simulink model "RS_O_yalmip"  (R2016b)
settings: Solver=ode1  StartTime=0.0  StopTime=T  FixedStep=1e-4  MaxStep=1e-3  RelTol=1e-6  EnableMultiTasking=on
InitFcn:
  | RS_O_script;
values from neighbouring files (symbols this model uses):
  C1 = 1e-9    (= 1e-09)    [Dati_MPC.m]
  C2 = 1e-9    (= 1e-09)    [Dati_MPC.m]
  Cext_Bp1 = Ce_Bp1*np_Bp1/ns_Bp1    (= 35750)    [Dati_MPC.m]
  Cext_Bp2 = Ce_Bp2*np_Bp2/ns_Bp2    (= 35750)    [Dati_MPC.m]
  Cext_BpM = Ce_BpM*np_BpM/ns_BpM    (= 68250)    [Dati_MPC.m]
  Cin_Bp1 = Ci_Bp1*np_Bp1/ns_Bp1    (= 16500)    [Dati_MPC.m]
  Cin_Bp2 = Ci_Bp2*np_Bp2/ns_Bp2    (= 16500)    [Dati_MPC.m]
  Cin_BpM = Ci_BpM*np_BpM/ns_BpM    (= 31500)    [Dati_MPC.m]
  Cint = 18e-3    (= 0.018)    [Dati_MPC.m]
  f = 50    [Dati_rete.m]
  ft_F = 10    [Dati_MPC.m]
  I_u = 0.1    [Dati_MPC.m]
  ki_PLL = w_t/Vd*(-w_t+sqrt(2*w_t^2-Vd^2*kp_PLL^2))    [Dati_MPC.m]
  kp_PLL = 0.9*kp_PLL_max    [Dati_MPC.m]
  MPCpar = struct    [Dati_MPC.m]    (also in Initialization.m)
  netdata = struct    [Dati_rete.m]
  P1 = 750e3    (= 750000)    [RS_O_script.m]
  P1v = 500e3    (= 500000)    [RS_O_script.m]
  P2 = 750e3    (= 750000)    [RS_O_script.m]
  P2v = 250e3    (= 250000)    [RS_O_script.m]
  P_u = 0.005    [Dati_MPC.m]
  Ppv1 = 500e3    (= 500000)    [Dati_MPC.m]
  Ppv2 = 850e3    (= 850000)    [Dati_MPC.m]
  Q1 = 350e3    (= 350000)    [RS_O_script.m]
  Q1v = 250e3    (= 250000)    [RS_O_script.m]
  Q2 = 300e3    (= 300000)    [RS_O_script.m]
  Q2v = 250e3    (= 250000)    [RS_O_script.m]
  Qbat1 = 50e3    (= 50000)    [Dati_MPC.m]
  Qbat2 = 50e3    (= 50000)    [Dati_MPC.m]
  Rext_Bp1 = Re_Bp1*ns_Bp1/np_Bp1    (= 0.0154545454545)    [Dati_MPC.m]
  Rext_Bp2 = Re_Bp2*ns_Bp2/np_Bp2    (= 0.0154545454545)    [Dati_MPC.m]
  Rext_BpM = Re_BpM*ns_BpM/np_BpM    (= 0.00809523809524)    [Dati_MPC.m]
  Rin_Bp1 = Ri_Bp1*ns_Bp1/np_Bp1    (= 0.363636363636)    [Dati_MPC.m]
  Rin_Bp2 = Ri_Bp2*ns_Bp2/np_Bp2    (= 0.363636363636)    [Dati_MPC.m]
  Rin_BpM = Ri_BpM*ns_BpM/np_BpM    (= 0.190476190476)    [Dati_MPC.m]
  SOC_10 = (Vbat1-Vbat1_min)/(Vbat1_max-Vbat1_min)    (= 0.625)    [Dati_MPC.m]
  SOC_20 = (Vbat2-Vbat2_min)/(Vbat2_max-Vbat2_min)    (= 0.625)    [Dati_MPC.m]
  SOC_M0 = (VbatM-VbatM_min)/(VbatM_max-VbatM_min)    (= 0.625)    [Dati_MPC.m]
  Srif = 1e6    (= 1000000)    [Dati_rete.m]
  t1 = 50    [RS_O_script.m]
  t2 = 110    [RS_O_script.m]
  t3 = 170    [RS_O_script.m]
  t_start_MPC = 10    [RS_O_script.m]
  tPLL = 2    [RS_O_script.m]
  Vbat1_max = 1.2*Vbat1_min    (= 480)    [Dati_MPC.m]
  Vbat1_min = 400    [Dati_MPC.m]
  Vbat2_max = 1.2*Vbat2_min    (= 480)    [Dati_MPC.m]
  Vbat2_min = 400    [Dati_MPC.m]
  VbatM_max = 1.2*VbatM_min    (= 480)    [Dati_MPC.m]
  VbatM_min = 400    [Dati_MPC.m]
  Vdc_1 = 800    [Dati_MPC.m]
  Vdc_2 = 800    [Dati_MPC.m]
  Vdc_M = 800    [Dati_MPC.m]
  Vrif_M = sqrt(2)/sqrt(3)*20e3    [Dati_MPC.m]
  Zrif = Vrif^2/Srif    (= 400)    [Dati_rete.m]
undefined symbols (not defined in the file or in its folder): Cfsc, Csc, j, L2, Lf, magnitude, Rc, Rint, Rsc
libraries: powerlib x87, powerlib_meascontrol x58, simulink x2
(part 1 of 3)
settings Model: SimulationMode=accelerator  Creator=10390222  LastModifiedBy=AlessioLaBella
settings SolverCC: ZeroCrossControl=EnableAll  SolverResetMethod=Robust
settings DataIOCC: LimitDataPoints=on
settings OptimizationCC: LifeSpan=inf
settings DebuggingCC: AllowSymbolicDim=off  SFUnexpectedBacktrackingDiag=warning  SFNoUnconditionalDefaultTransitionDiag=warning  SFExecutionAtInitializationDiag=none
settings ModelReferenceCC: PropagateSignalLabelsOutOfModel=off
settings GRTTargetCC: TargetLangStandard=C89/C90 (ANSI)
settings ConfigComp: CovMetricSettings=dw  CovHtmlReporting=on  CovSaveCumulativeToWorkspaceVar=on  CovSaveSingleToWorkspaceVar=on  CovExternalEMLEnable=off

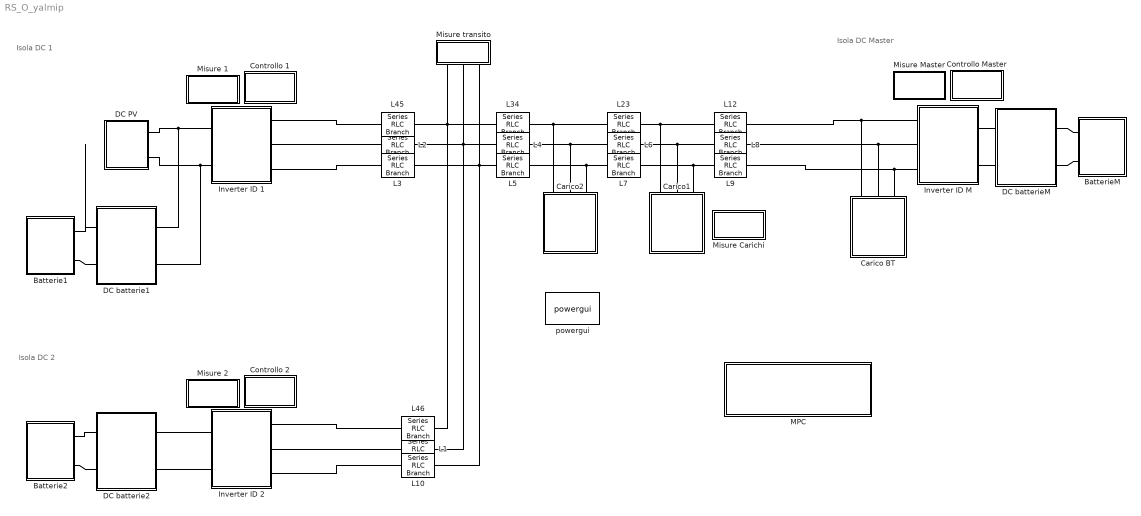
== system RS_O_yalmip ==
  note: Isola DC Master
  note: Isola DC 1
  note: Isola DC 2
  Batterie1 : Subsystem
  Batterie2 : Subsystem
  BatterieM : Subsystem
  Carico BT : Subsystem
  Carico1 : Subsystem
  Carico2 : Subsystem
  Controllo 1 : Subsystem
  Controllo 2 : Subsystem
  Controllo Master : Subsystem
  DC PV : Subsystem
  DC batterie1 : Subsystem
  DC batterie2 : Subsystem
  DC batterieM : Subsystem
  Inverter ID 1 : Subsystem
  Inverter ID 2 : Subsystem
  Inverter ID M : Subsystem
  L1 : powerlib/Elements/Series RLC Branch  LConnTagsString=__new0  RConnTagsString=__new0  BranchType=RL  Resistance=netdata.R(5)*Zrif  Inductance=netdata.L(5)*Zrif  SetiL0=off  InitialCurrent=0  Capacitance=1e-6  Setx0=off  InitialVoltage=0  Measurements=None
  L10 : powerlib/Elements/Series RLC Branch  LConnTagsString=__new0  RConnTagsString=__new0  BranchType=RL  Resistance=netdata.R(5)*Zrif  Inductance=netdata.L(5)*Zrif  SetiL0=off  InitialCurrent=0  Capacitance=1e-6  Setx0=off  InitialVoltage=0  Measurements=None
  L12 : powerlib/Elements/Series RLC Branch  LConnTagsString=__new0  RConnTagsString=__new0  BranchType=RL  Resistance=netdata.R(1)*Zrif  Inductance=netdata.L(1)*Zrif  SetiL0=off  InitialCurrent=0  Capacitance=1e-6  Setx0=off  InitialVoltage=0  Measurements=None
  L2 : powerlib/Elements/Series RLC Branch  LConnTagsString=__new0  RConnTagsString=__new0  BranchType=RL  Resistance=netdata.R(4)*Zrif  Inductance=netdata.L(4)*Zrif  SetiL0=off  InitialCurrent=0  Capacitance=1e-6  Setx0=off  InitialVoltage=0  Measurements=None
  L23 : powerlib/Elements/Series RLC Branch  LConnTagsString=__new0  RConnTagsString=__new0  BranchType=RL  Resistance=netdata.R(2)*Zrif  Inductance=netdata.L(2)*Zrif  SetiL0=off  InitialCurrent=0  Capacitance=1e-6  Setx0=off  InitialVoltage=0  Measurements=None
  L3 : powerlib/Elements/Series RLC Branch  LConnTagsString=__new0  RConnTagsString=__new0  BranchType=RL  Resistance=netdata.R(4)*Zrif  Inductance=netdata.L(4)*Zrif  SetiL0=off  InitialCurrent=0  Capacitance=1e-6  Setx0=off  InitialVoltage=0  Measurements=None
  L34 : powerlib/Elements/Series RLC Branch  LConnTagsString=__new0  RConnTagsString=__new0  BranchType=RL  Resistance=netdata.R(3)*Zrif  Inductance=netdata.L(3)*Zrif  SetiL0=off  InitialCurrent=0  Capacitance=1e-6  Setx0=off  InitialVoltage=0  Measurements=None
  L4 : powerlib/Elements/Series RLC Branch  LConnTagsString=__new0  RConnTagsString=__new0  BranchType=RL  Resistance=netdata.R(3)*Zrif  Inductance=netdata.L(3)*Zrif  SetiL0=off  InitialCurrent=0  Capacitance=1e-6  Setx0=off  InitialVoltage=0  Measurements=None
  L45 : powerlib/Elements/Series RLC Branch  LConnTagsString=__new0  RConnTagsString=__new0  BranchType=RL  Resistance=netdata.R(4)*Zrif  Inductance=netdata.L(4)*Zrif  SetiL0=off  InitialCurrent=0  Capacitance=1e-6  Setx0=off  InitialVoltage=0  Measurements=None
  L46 : powerlib/Elements/Series RLC Branch  LConnTagsString=__new0  RConnTagsString=__new0  BranchType=RL  Resistance=netdata.R(5)*Zrif  Inductance=netdata.L(5)*Zrif  SetiL0=off  InitialCurrent=0  Capacitance=1e-6  Setx0=off  InitialVoltage=0  Measurements=None
  L5 : powerlib/Elements/Series RLC Branch  LConnTagsString=__new0  RConnTagsString=__new0  BranchType=RL  Resistance=netdata.R(3)*Zrif  Inductance=netdata.L(3)*Zrif  SetiL0=off  InitialCurrent=0  Capacitance=1e-6  Setx0=off  InitialVoltage=0  Measurements=None
  L6 : powerlib/Elements/Series RLC Branch  LConnTagsString=__new0  RConnTagsString=__new0  BranchType=RL  Resistance=netdata.R(2)*Zrif  Inductance=netdata.L(2)*Zrif  SetiL0=off  InitialCurrent=0  Capacitance=1e-6  Setx0=off  InitialVoltage=0  Measurements=None
  L7 : powerlib/Elements/Series RLC Branch  LConnTagsString=__new0  RConnTagsString=__new0  BranchType=RL  Resistance=netdata.R(2)*Zrif  Inductance=netdata.L(2)*Zrif  SetiL0=off  InitialCurrent=0  Capacitance=1e-6  Setx0=off  InitialVoltage=0  Measurements=None
  L8 : powerlib/Elements/Series RLC Branch  LConnTagsString=__new0  RConnTagsString=__new0  BranchType=RL  Resistance=netdata.R(1)*Zrif  Inductance=netdata.L(1)*Zrif  SetiL0=off  InitialCurrent=0  Capacitance=1e-6  Setx0=off  InitialVoltage=0  Measurements=None
  L9 : powerlib/Elements/Series RLC Branch  LConnTagsString=__new0  RConnTagsString=__new0  BranchType=RL  Resistance=netdata.R(1)*Zrif  Inductance=netdata.L(1)*Zrif  SetiL0=off  InitialCurrent=0  Capacitance=1e-6  Setx0=off  InitialVoltage=0  Measurements=None
  MPC : Subsystem
  Misure 1 : Subsystem
  Misure 2 : Subsystem
  Misure Carichi : Subsystem
  Misure Master : Subsystem
  Misure transito : Subsystem
  powergui : powerlib/powergui  Priority=1  SimulationMode=Discrete  SolverType=Backward Euler  SampleTime=1e-4  frequency=60  SPID=off  DisableSnubberDevices=off  DisableRonSwitches=off  DisableVfSwitches=off  SwTol=0  DisplayEquations=off  Interpol=off  ExternalGateDelay=off  methode=off  Ts=10  FunctionMessages=off  echomessages=off  HookPort=off  EnableUseOfTLC=off  x0status=blocks  frequencyindice=0  Pbase=100e6  ErrMax=1e-4  Iterations=50  UnitsV=kV  UnitsW=MW  buscounter=0  RestoreLinks=warning  ResistiveCurrentMeasurement=off  Frange=[0:2:500]  Ylog=off  Xlog=on  ShowGrid=off  save=off  variable=ZData  structure=If  ZoomFFT=off  StartTime=1  cycles=10  DisplayStyle=1  fundamental=50  FreqAxis=off  MaxFrequency=200  frequencyindicesteady=1  RmsSteady=1  display=off
  connections:
  Carico1/LConn2 -- L6/RConn1 -- L8/LConn1
  L12/LConn1 -- L23/RConn1 -- Carico1/LConn1
  Carico1/LConn3 -- L7/RConn1 -- L9/LConn1
  Carico2/LConn2 -- L4/RConn1 -- L6/LConn1
  Carico2/LConn1 -- L23/LConn1 -- L34/RConn1
  Carico2/LConn3 -- L5/RConn1 -- L7/LConn1
  L34/LConn1 -- L45/RConn1 -- Misure transito/LConn1 -- L46/RConn1
  Misure transito/LConn2 -- L1/RConn1 -- L2/RConn1 -- L4/LConn1
  Misure transito/LConn3 -- L10/RConn1 -- L3/RConn1 -- L5/LConn1
  Inverter ID 1/RConn1 -- L45/LConn1
  L3/LConn1 -- Inverter ID 1/RConn3
  L2/LConn1 -- Inverter ID 1/RConn2
  L1/LConn1 -- Inverter ID 2/RConn2
  Inverter ID 2/RConn1 -- L46/LConn1
  Inverter ID 2/RConn3 -- L10/LConn1
  DC batterie1/LConn2 -- Batterie1/RConn2
  DC batterie1/LConn1 -- Batterie1/RConn1
  DC PV/RConn1 -- DC batterie1/RConn1 -- Inverter ID 1/LConn1
  DC PV/RConn2 -- DC batterie1/RConn2 -- Inverter ID 1/LConn2
  DC batterie2/RConn2 -- Inverter ID 2/LConn2
  DC batterie2/RConn1 -- Inverter ID 2/LConn1
  DC batterieM/RConn1 -- Inverter ID M/LConn1
  Inverter ID M/RConn1 -- L12/RConn1 -- Carico BT/LConn1
  Inverter ID M/RConn2 -- L8/RConn1 -- Carico BT/LConn2
  Inverter ID M/RConn3 -- L9/RConn1 -- Carico BT/LConn3
  DC batterie2/LConn1 -- Batterie2/RConn1
  DC batterie2/LConn2 -- Batterie2/RConn2
  DC batterieM/LConn1 -- BatterieM/RConn1
  DC batterieM/LConn2 -- BatterieM/RConn2
  DC batterieM/RConn2 -- Inverter ID M/LConn2

== system RS_O_yalmip/Batterie1 ==
  Cext : powerlib/Elements/Series RLC Branch  LConnTagsString=__new0  RConnTagsString=__new0  BranchType=C  Resistance=Rint  Inductance=0  SetiL0=off  InitialCurrent=0  Capacitance=Cext_Bp1  Setx0=on  InitialVoltage=Vbat1  Measurements=None
  Cin : powerlib/Elements/Series RLC Branch  LConnTagsString=__new0  RConnTagsString=__new0  BranchType=C  Resistance=Rsc  Inductance=L2  SetiL0=on  InitialCurrent=0  Capacitance=Cin_Bp1  Setx0=on  InitialVoltage=Vbat1  Measurements=None
  Rext : powerlib/Elements/Series RLC Branch  LConnTagsString=__new0  RConnTagsString=__new0  BranchType=R  Resistance=Rext_Bp1  Inductance=0  SetiL0=off  InitialCurrent=0  Capacitance=Cfsc  Setx0=on  InitialVoltage=Vsc  Measurements=None
  Rin : powerlib/Elements/Series RLC Branch  LConnTagsString=__new0  RConnTagsString=__new0  BranchType=R  Resistance=Rin_Bp1  Inductance=L2  SetiL0=on  InitialCurrent=0  Capacitance=Csc  Setx0=on  InitialVoltage=Vsc  Measurements=None
  bat + : PMIOPort  Port=1  Side=Right
  bat - : PMIOPort  Port=2  Side=Right
  connections:
  bat +/RConn1 -- Rext/RConn1
  Rext/LConn1 -- Cext/LConn1 -- Rin/RConn1
  Cin/LConn1 -- Rin/LConn1
  Cin/RConn1 -- bat -/RConn1 -- Cext/RConn1

== system RS_O_yalmip/Batterie2 ==
  Cext : powerlib/Elements/Series RLC Branch  LConnTagsString=__new0  RConnTagsString=__new0  BranchType=C  Resistance=Rint  Inductance=0  SetiL0=off  InitialCurrent=0  Capacitance=Cext_Bp2  Setx0=on  InitialVoltage=Vbat2  Measurements=None
  Cin : powerlib/Elements/Series RLC Branch  LConnTagsString=__new0  RConnTagsString=__new0  BranchType=C  Resistance=Rsc  Inductance=L2  SetiL0=on  InitialCurrent=0  Capacitance=Cin_Bp2  Setx0=on  InitialVoltage=Vbat2  Measurements=None
  Rext : powerlib/Elements/Series RLC Branch  LConnTagsString=__new0  RConnTagsString=__new0  BranchType=R  Resistance=Rext_Bp2  Inductance=0  SetiL0=off  InitialCurrent=0  Capacitance=Cfsc  Setx0=on  InitialVoltage=Vsc  Measurements=None
  Rin : powerlib/Elements/Series RLC Branch  LConnTagsString=__new0  RConnTagsString=__new0  BranchType=R  Resistance=Rin_Bp2  Inductance=L2  SetiL0=on  InitialCurrent=0  Capacitance=Csc  Setx0=on  InitialVoltage=Vsc  Measurements=None
  bat + : PMIOPort  Port=1  Side=Right
  bat - : PMIOPort  Port=2  Side=Right
  connections:
  Cext/RConn1 -- bat -/RConn1 -- Cin/RConn1
  Cin/LConn1 -- Rin/LConn1
  Rin/RConn1 -- Cext/LConn1 -- Rext/LConn1
  bat +/RConn1 -- Rext/RConn1

== system RS_O_yalmip/BatterieM ==
  Cext : powerlib/Elements/Series RLC Branch  LConnTagsString=__new0  RConnTagsString=__new0  BranchType=C  Resistance=Rint  Inductance=0  SetiL0=off  InitialCurrent=0  Capacitance=Cext_BpM  Setx0=on  InitialVoltage=VbatM  Measurements=None
  Cin : powerlib/Elements/Series RLC Branch  LConnTagsString=__new0  RConnTagsString=__new0  BranchType=C  Resistance=Rsc  Inductance=L2  SetiL0=on  InitialCurrent=0  Capacitance=Cin_BpM  Setx0=on  InitialVoltage=VbatM  Measurements=None
  Rext : powerlib/Elements/Series RLC Branch  LConnTagsString=__new0  RConnTagsString=__new0  BranchType=R  Resistance=Rext_BpM  Inductance=0  SetiL0=off  InitialCurrent=0  Capacitance=Cfsc  Setx0=on  InitialVoltage=Vsc  Measurements=None
  Rin : powerlib/Elements/Series RLC Branch  LConnTagsString=__new0  RConnTagsString=__new0  BranchType=R  Resistance=Rin_BpM  Inductance=L2  SetiL0=on  InitialCurrent=0  Capacitance=Csc  Setx0=on  InitialVoltage=Vsc  Measurements=None
  bat + : PMIOPort  Port=1  Side=Right
  bat - : PMIOPort  Port=2  Side=Right
  connections:
  Cext/RConn1 -- bat -/RConn1 -- Cin/RConn1
  Cin/LConn1 -- Rin/LConn1
  Rin/RConn1 -- Cext/LConn1 -- Rext/LConn1
  bat +/RConn1 -- Rext/RConn1

== system RS_O_yalmip/Carico BT ==
  Carico BT : powerlib/Elements/Three-Phase Series RLC Load  LConnTagsString=A|B|C  Configuration=Y (floating)  NominalVoltage=20e3  Vabc=[1e3 1e3 1e3]  Vabcp=[1e3 1e3 1e3]  NominalFrequency=50  UnbalancedPower=off  ActivePower=Pbt  InductivePower=Qbt  CapacitivePower=0  Pabc=[10e3 9e3 11e3]  QLabc=[100 90 110]  QCabc=[100 90 110]  Pabcp=[10e3 9e3 11e3]  QLabcp=[100 90 110]  QCabcp=[100 90 110]  Measurements=None  LoadType=constant Z
  Three-Phase V-I Measurement2 : powerlib/Measurements/Three-Phase V-I Measurement  VoltageMeasurement=phase-to-phase  SetLabelV=off  LabelV=Vabc  Vpu=off  VpuLL=off  CurrentMeasurement=yes  SetLabelI=off  LabelI=Iabc  Ipu=off  Pbase=100e6  Vbase=500e3  OutputType=Complex  PhasorSimulation=off  PSBequivalent=0
  V,I carico BT : Scope  NumInputPorts=2
  A : PMIOPort  Port=1  Side=Left
  B : PMIOPort  Port=2  Side=Left
  C : PMIOPort  Port=3  Side=Left
  wires:
  Three-Phase V-I Measurement2/1 -> V,I carico BT/1
  Three-Phase V-I Measurement2/2 -> V,I carico BT/2
  connections:
  Three-Phase V-I Measurement2/LConn1 -- A/RConn1
  Three-Phase V-I Measurement2/LConn2 -- B/RConn1
  Three-Phase V-I Measurement2/LConn3 -- C/RConn1
  Carico BT/LConn2 -- Three-Phase V-I Measurement2/RConn2
  Carico BT/LConn1 -- Three-Phase V-I Measurement2/RConn1
  Carico BT/LConn3 -- Three-Phase V-I Measurement2/RConn3

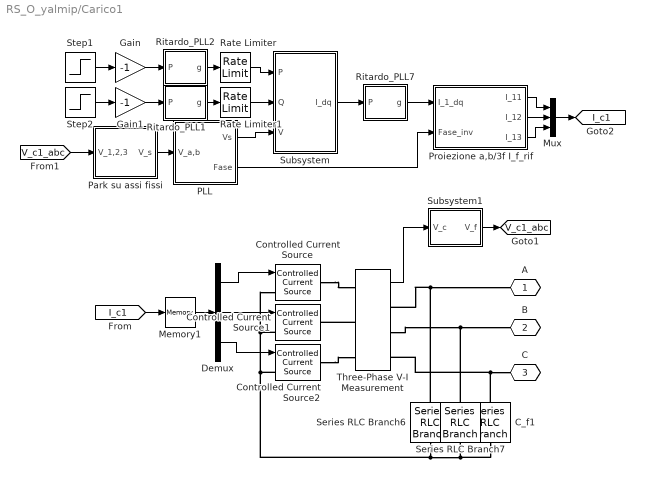
== system RS_O_yalmip/Carico1 ==
  C_f1 : powerlib/Elements/Series RLC Branch  LConnTagsString=__new0  RConnTagsString=__new0  BranchType=C  Resistance=Rc  Inductance=Lf  SetiL0=off  InitialCurrent=0  Capacitance=C1  Setx0=off  InitialVoltage=0  Measurements=None
  Controlled Current Source : powerlib/Electrical Sources/Controlled Current Source  Initialize=on  Source_Type=AC  Amplitude=0  Phase=0  Frequency=0  Measurements=None
  Controlled Current Source1 : powerlib/Electrical Sources/Controlled Current Source  Initialize=on  Source_Type=AC  Amplitude=0  Phase=0  Frequency=0  Measurements=None
  Controlled Current Source2 : powerlib/Electrical Sources/Controlled Current Source  Initialize=on  Source_Type=AC  Amplitude=0  Phase=0  Frequency=0  Measurements=None
  Demux : Demux  Outputs=3
  Gain : Gain  Gain=-1
  Gain1 : Gain  Gain=-1
  Memory1 : Memory
  Mux : Mux  Inputs=3
  PLL : Subsystem
  Park su assi fissi : Subsystem
  Proiezione a,b/3f I_f_rif : Subsystem
  Rate Limiter : RateLimiter  RisingSlewLimit=1e6  FallingSlewLimit=-1e6  SampleTimeMode=inherited
  Rate Limiter1 : RateLimiter  RisingSlewLimit=1e6  FallingSlewLimit=-1e6  SampleTimeMode=inherited
  Ritardo_PLL1 : Subsystem
  Ritardo_PLL2 : Subsystem
  Ritardo_PLL7 : Subsystem
  Series RLC Branch6 : powerlib/Elements/Series RLC Branch  LConnTagsString=__new0  RConnTagsString=__new0  BranchType=C  Resistance=Rc  Inductance=Lf  SetiL0=off  InitialCurrent=0  Capacitance=C1  Setx0=off  InitialVoltage=0  Measurements=None
  Series RLC Branch7 : powerlib/Elements/Series RLC Branch  LConnTagsString=__new0  RConnTagsString=__new0  BranchType=C  Resistance=Rc  Inductance=Lf  SetiL0=off  InitialCurrent=0  Capacitance=C1  Setx0=off  InitialVoltage=0  Measurements=None
  Step1 : Step  Time=t1  Before=P1  After=P1+P1v  SampleTime=0
  Step2 : Step  Time=t1  Before=Q1  After=Q1+Q1v  SampleTime=0
  Subsystem : Subsystem
  Subsystem1 : Subsystem
  Three-Phase V-I Measurement : powerlib/Measurements/Three-Phase V-I Measurement  VoltageMeasurement=phase-to-phase  SetLabelV=off  LabelV=Vabc  Vpu=off  VpuLL=off  CurrentMeasurement=no  SetLabelI=off  LabelI=Iabc  Ipu=off  Pbase=100e6  Vbase=500e3  OutputType=Complex  PhasorSimulation=off  PSBequivalent=0
  A : PMIOPort  Port=1  Side=Left
  B : PMIOPort  Port=2  Side=Left
  C : PMIOPort  Port=3  Side=Left
  tag scope: I_c1=global, V_c1_abc=global
  wires:
  Three-Phase V-I Measurement/1 -> Subsystem1/1(V_c)
  Demux/2 -> Controlled Current Source1/1
  Demux/3 -> Controlled Current Source2/1
  Demux/1 -> Controlled Current Source/1
  [I_c1] -> Memory1/1
  Memory1/1 -> Demux/1
  Subsystem1/1(V_f) -> [V_c1_abc]
  Proiezione a,b/3f I_f_rif/3(I_13) -> Mux/3
  Subsystem/1(I_dq) -> Ritardo_PLL7/1(P)
  Proiezione a,b/3f I_f_rif/2(I_12) -> Mux/2
  Proiezione a,b/3f I_f_rif/1(I_11) -> Mux/1
  Mux/1 -> [I_c1]
  PLL/2(Fase) -> Proiezione a,b/3f I_f_rif/2(Fase_inv)
  [V_c1_abc] -> Park su assi fissi/1(V_1,2,3)
  Ritardo_PLL7/1(g) -> Proiezione a,b/3f I_f_rif/1(I_1_dq)
  Park su assi fissi/1(V_s) -> PLL/1(V_a,b)
  PLL/1(Vs) -> Subsystem/3(V)
  Rate Limiter/1 -> Subsystem/1(P)
  Rate Limiter1/1 -> Subsystem/2(Q)
  Ritardo_PLL1/1(g) -> Rate Limiter1/1
  Ritardo_PLL2/1(g) -> Rate Limiter/1
  Gain1/1 -> Ritardo_PLL1/1(P)
  Gain/1 -> Ritardo_PLL2/1(P)
  Step2/1 -> Gain1/1
  Step1/1 -> Gain/1
  connections:
  Series RLC Branch7/RConn1 -- C_f1/RConn1 -- Series RLC Branch6/RConn1 -- Controlled Current Source2/LConn1 -- Controlled Current Source1/LConn1 -- Controlled Current Source/LConn1
  Three-Phase V-I Measurement/RConn2 -- B/RConn1 -- Series RLC Branch7/LConn1
  Series RLC Branch6/LConn1 -- Three-Phase V-I Measurement/RConn1 -- A/RConn1
  C_f1/LConn1 -- C/RConn1 -- Three-Phase V-I Measurement/RConn3
  Controlled Current Source/RConn1 -- Three-Phase V-I Measurement/LConn1
  Controlled Current Source2/RConn1 -- Three-Phase V-I Measurement/LConn3
  Three-Phase V-I Measurement/LConn2 -- Controlled Current Source1/RConn1

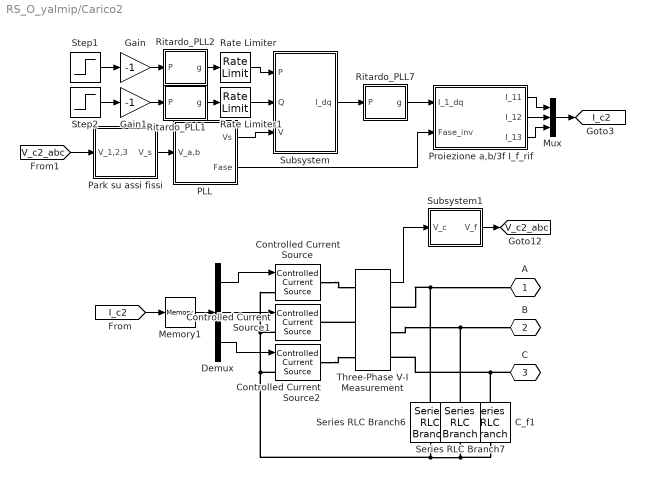
== system RS_O_yalmip/Carico2 ==
  C_f1 : powerlib/Elements/Series RLC Branch  LConnTagsString=__new0  RConnTagsString=__new0  BranchType=C  Resistance=Rc  Inductance=Lf  SetiL0=off  InitialCurrent=0  Capacitance=C1  Setx0=off  InitialVoltage=0  Measurements=None
  Controlled Current Source : powerlib/Electrical Sources/Controlled Current Source  Initialize=on  Source_Type=AC  Amplitude=0  Phase=0  Frequency=0  Measurements=None
  Controlled Current Source1 : powerlib/Electrical Sources/Controlled Current Source  Initialize=on  Source_Type=AC  Amplitude=0  Phase=0  Frequency=0  Measurements=None
  Controlled Current Source2 : powerlib/Electrical Sources/Controlled Current Source  Initialize=on  Source_Type=AC  Amplitude=0  Phase=0  Frequency=0  Measurements=None
  Demux : Demux  Outputs=3
  Gain : Gain  Gain=-1
  Gain1 : Gain  Gain=-1
  Memory1 : Memory
  Mux : Mux  Inputs=3
  PLL : Subsystem
  Park su assi fissi : Subsystem
  Proiezione a,b/3f I_f_rif : Subsystem
  Rate Limiter : RateLimiter  RisingSlewLimit=1e6  FallingSlewLimit=-1e6  SampleTimeMode=inherited
  Rate Limiter1 : RateLimiter  RisingSlewLimit=1e6  FallingSlewLimit=-1e6  SampleTimeMode=inherited
  Ritardo_PLL1 : Subsystem
  Ritardo_PLL2 : Subsystem
  Ritardo_PLL7 : Subsystem
  Series RLC Branch6 : powerlib/Elements/Series RLC Branch  LConnTagsString=__new0  RConnTagsString=__new0  BranchType=C  Resistance=Rc  Inductance=Lf  SetiL0=off  InitialCurrent=0  Capacitance=C1  Setx0=off  InitialVoltage=0  Measurements=None
  Series RLC Branch7 : powerlib/Elements/Series RLC Branch  LConnTagsString=__new0  RConnTagsString=__new0  BranchType=C  Resistance=Rc  Inductance=Lf  SetiL0=off  InitialCurrent=0  Capacitance=C1  Setx0=off  InitialVoltage=0  Measurements=None
  Step1 : Step  Time=t2  Before=P2  After=P2+P2v  SampleTime=0
  Step2 : Step  Time=t2  Before=Q2  After=Q2+Q2v  SampleTime=0
  Subsystem : Subsystem
  Subsystem1 : Subsystem
  Three-Phase V-I Measurement : powerlib/Measurements/Three-Phase V-I Measurement  VoltageMeasurement=phase-to-phase  SetLabelV=off  LabelV=Vabc  Vpu=off  VpuLL=off  CurrentMeasurement=no  SetLabelI=off  LabelI=Iabc  Ipu=off  Pbase=100e6  Vbase=500e3  OutputType=Complex  PhasorSimulation=off  PSBequivalent=0
  A : PMIOPort  Port=1  Side=Left
  B : PMIOPort  Port=2  Side=Left
  C : PMIOPort  Port=3  Side=Left
  tag scope: I_c2=global, V_c2_abc=global
  wires:
  Three-Phase V-I Measurement/1 -> Subsystem1/1(V_c)
  Demux/2 -> Controlled Current Source1/1
  Demux/3 -> Controlled Current Source2/1
  Demux/1 -> Controlled Current Source/1
  [I_c2] -> Memory1/1
  Memory1/1 -> Demux/1
  Subsystem1/1(V_f) -> [V_c2_abc]
  Proiezione a,b/3f I_f_rif/3(I_13) -> Mux/3
  Subsystem/1(I_dq) -> Ritardo_PLL7/1(P)
  Proiezione a,b/3f I_f_rif/2(I_12) -> Mux/2
  Proiezione a,b/3f I_f_rif/1(I_11) -> Mux/1
  Mux/1 -> [I_c2]
  PLL/2(Fase) -> Proiezione a,b/3f I_f_rif/2(Fase_inv)
  [V_c2_abc] -> Park su assi fissi/1(V_1,2,3)
  Ritardo_PLL7/1(g) -> Proiezione a,b/3f I_f_rif/1(I_1_dq)
  Park su assi fissi/1(V_s) -> PLL/1(V_a,b)
  PLL/1(Vs) -> Subsystem/3(V)
  Rate Limiter/1 -> Subsystem/1(P)
  Rate Limiter1/1 -> Subsystem/2(Q)
  Ritardo_PLL1/1(g) -> Rate Limiter1/1
  Ritardo_PLL2/1(g) -> Rate Limiter/1
  Step1/1 -> Gain/1
  Step2/1 -> Gain1/1
  Gain/1 -> Ritardo_PLL2/1(P)
  Gain1/1 -> Ritardo_PLL1/1(P)
  connections:
  Series RLC Branch7/RConn1 -- C_f1/RConn1 -- Series RLC Branch6/RConn1 -- Controlled Current Source2/LConn1 -- Controlled Current Source1/LConn1 -- Controlled Current Source/LConn1
  Series RLC Branch7/LConn1 -- Three-Phase V-I Measurement/RConn2 -- B/RConn1
  Three-Phase V-I Measurement/RConn1 -- A/RConn1 -- Series RLC Branch6/LConn1
  Controlled Current Source2/RConn1 -- Three-Phase V-I Measurement/LConn3
  Controlled Current Source/RConn1 -- Three-Phase V-I Measurement/LConn1
  Three-Phase V-I Measurement/LConn2 -- Controlled Current Source1/RConn1
  C_f1/LConn1 -- C/RConn1 -- Three-Phase V-I Measurement/RConn3

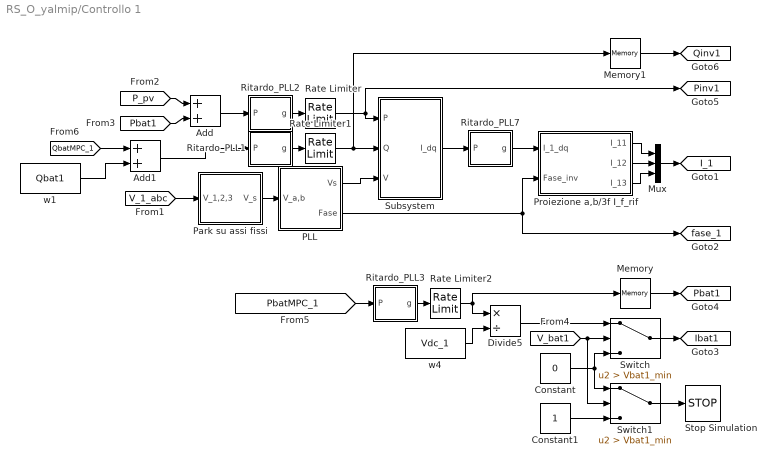
== system RS_O_yalmip/Controllo 1 ==
  Add : Sum
  Add1 : Sum
  Constant : Constant  Value=0
  Constant1 : Constant
  Divide5 : Product  Inputs=*/
  Memory : Memory
  Memory1 : Memory
  Mux : Mux  Inputs=3
  PLL : Subsystem
  Park su assi fissi : Subsystem
  Proiezione a,b/3f I_f_rif : Subsystem
  Rate Limiter : RateLimiter  RisingSlewLimit=1e8  FallingSlewLimit=-1e8  SampleTimeMode=inherited
  Rate Limiter1 : RateLimiter  RisingSlewLimit=1e8  FallingSlewLimit=-1e8  SampleTimeMode=inherited
  Rate Limiter2 : RateLimiter  RisingSlewLimit=1e8  FallingSlewLimit=-1e8  SampleTimeMode=inherited
  Ritardo_PLL1 : Subsystem
  Ritardo_PLL2 : Subsystem
  Ritardo_PLL3 : Subsystem
  Ritardo_PLL7 : Subsystem
  Stop Simulation : Stop
  Subsystem : Subsystem
  Switch : Switch  Criteria=u2 > Threshold  Threshold=Vbat1_min
  Switch1 : Switch  Criteria=u2 > Threshold  Threshold=Vbat1_min
  w1 : Constant  Value=Qbat1
  w4 : Constant  Value=Vdc_1
  tag scope: I_1=global, Ibat1=global, Pbat1=global, Pinv1=global, Qinv1=global, fase_1=global
  wires:
  Proiezione a,b/3f I_f_rif/3(I_13) -> Mux/3
  Subsystem/1(I_dq) -> Ritardo_PLL7/1(P)
  Proiezione a,b/3f I_f_rif/2(I_12) -> Mux/2
  Proiezione a,b/3f I_f_rif/1(I_11) -> Mux/1
  Mux/1 -> [I_1]
  PLL/2(Fase) -> Proiezione a,b/3f I_f_rif/2(Fase_inv), [fase_1]
  Add1/1 -> Ritardo_PLL1/1(P)
  [V_1_abc] -> Park su assi fissi/1(V_1,2,3)
  Ritardo_PLL7/1(g) -> Proiezione a,b/3f I_f_rif/1(I_1_dq)
  Park su assi fissi/1(V_s) -> PLL/1(V_a,b)
  PLL/1(Vs) -> Subsystem/3(V)
  Rate Limiter1/1 -> Memory1/1, Subsystem/2(Q)
  Ritardo_PLL1/1(g) -> Rate Limiter1/1
  Ritardo_PLL2/1(g) -> Rate Limiter/1
  Rate Limiter2/1 -> Divide5/1, Memory/1
  w4/1 -> Divide5/2
  Ritardo_PLL3/1(g) -> Rate Limiter2/1
  [PbatMPC_1] -> Ritardo_PLL3/1(P)
  Add/1 -> Ritardo_PLL2/1(P)
  [P_pv] -> Add/1
  [Pbat1] -> Add/2
  Rate Limiter/1 -> [Pinv1], Subsystem/1(P)
  Switch/1 -> [Ibat1]
  Divide5/1 -> Switch/1
  [V_bat1] -> Switch/2, Switch1/2
  Constant/1 -> Switch1/1, Switch/3
  Constant1/1 -> Switch1/3
  Switch1/1 -> Stop Simulation/1
  Memory/1 -> [Pbat1]
  Memory1/1 -> [Qinv1]
  [QbatMPC_1] -> Add1/1
  w1/1 -> Add1/2

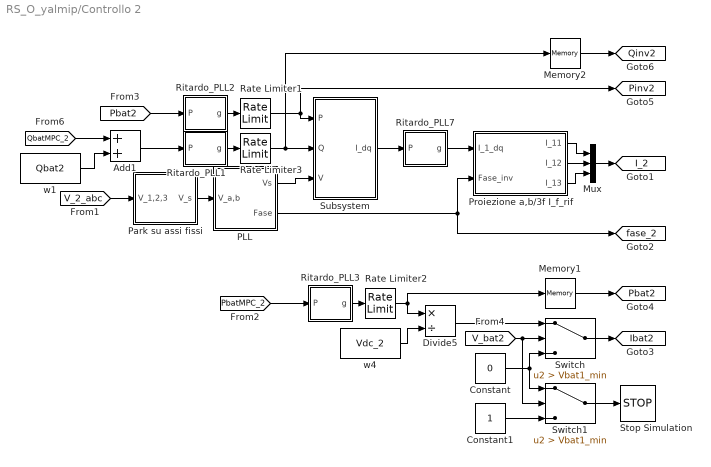
== system RS_O_yalmip/Controllo 2 ==
  Add1 : Sum
  Constant : Constant  Value=0
  Constant1 : Constant
  Divide5 : Product  Inputs=*/
  Memory1 : Memory
  Memory2 : Memory
  Mux : Mux  Inputs=3
  PLL : Subsystem
  Park su assi fissi : Subsystem
  Proiezione a,b/3f I_f_rif : Subsystem
  Rate Limiter1 : RateLimiter  RisingSlewLimit=1e8  FallingSlewLimit=-1e8  SampleTimeMode=inherited
  Rate Limiter2 : RateLimiter  RisingSlewLimit=1e8  FallingSlewLimit=-1e8  SampleTimeMode=inherited
  Rate Limiter3 : RateLimiter  RisingSlewLimit=1e8  FallingSlewLimit=-1e8  SampleTimeMode=inherited
  Ritardo_PLL1 : Subsystem
  Ritardo_PLL2 : Subsystem
  Ritardo_PLL3 : Subsystem
  Ritardo_PLL7 : Subsystem
  Stop Simulation : Stop
  Subsystem : Subsystem
  Switch : Switch  Criteria=u2 > Threshold  Threshold=Vbat1_min
  Switch1 : Switch  Criteria=u2 > Threshold  Threshold=Vbat1_min
  w1 : Constant  Value=Qbat2
  w4 : Constant  Value=Vdc_2
  tag scope: I_2=global, Ibat2=global, Pbat2=global, Pinv2=global, Qinv2=global, fase_2=global
  wires:
  Switch1/1 -> Stop Simulation/1
  Constant1/1 -> Switch1/3
  PLL/1(Vs) -> Subsystem/3(V)
  Add1/1 -> Ritardo_PLL1/1(P)
  Proiezione a,b/3f I_f_rif/3(I_13) -> Mux/3
  [V_2_abc] -> Park su assi fissi/1(V_1,2,3)
  Mux/1 -> [I_2]
  Switch/1 -> [Ibat2]
  [V_bat2] -> Switch/2, Switch1/2
  Divide5/1 -> Switch/1
  [PbatMPC_2] -> Ritardo_PLL3/1(P)
  [Pbat2] -> Ritardo_PLL2/1(P)
  w4/1 -> Divide5/2
  Ritardo_PLL3/1(g) -> Rate Limiter2/1
  Subsystem/1(I_dq) -> Ritardo_PLL7/1(P)
  Ritardo_PLL2/1(g) -> Rate Limiter1/1
  Ritardo_PLL1/1(g) -> Rate Limiter3/1
  Rate Limiter3/1 -> Memory2/1, Subsystem/2(Q)
  Rate Limiter2/1 -> Divide5/1, Memory1/1
  Constant/1 -> Switch1/1, Switch/3
  Ritardo_PLL7/1(g) -> Proiezione a,b/3f I_f_rif/1(I_1_dq)
  PLL/2(Fase) -> Proiezione a,b/3f I_f_rif/2(Fase_inv), [fase_2]
  Park su assi fissi/1(V_s) -> PLL/1(V_a,b)
  Proiezione a,b/3f I_f_rif/1(I_11) -> Mux/1
  Rate Limiter1/1 -> [Pinv2], Subsystem/1(P)
  Proiezione a,b/3f I_f_rif/2(I_12) -> Mux/2
  Memory1/1 -> [Pbat2]
  Memory2/1 -> [Qinv2]
  w1/1 -> Add1/2
  [QbatMPC_2] -> Add1/1

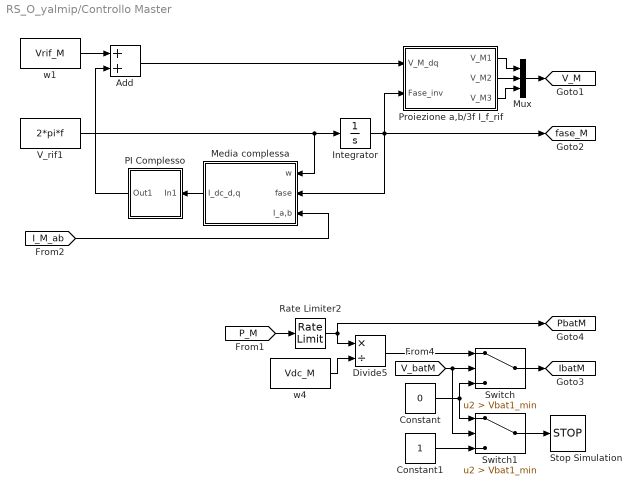
== system RS_O_yalmip/Controllo Master ==
  Add : Sum
  Constant : Constant  Value=0
  Constant1 : Constant
  Divide5 : Product  Inputs=*/
  Integrator : Integrator  UpperSaturationLimit=50  LowerSaturationLimit=-50  WrapState=on
  Media complessa : Subsystem
  Mux : Mux  Inputs=3
  PI Complesso : Subsystem
  Proiezione a,b/3f I_f_rif : Subsystem
  Rate Limiter2 : RateLimiter  RisingSlewLimit=1e6  FallingSlewLimit=-1e6  SampleTimeMode=inherited
  Stop Simulation : Stop
  Switch : Switch  Criteria=u2 > Threshold  Threshold=Vbat1_min
  Switch1 : Switch  Criteria=u2 > Threshold  Threshold=Vbat1_min
  V_rif1 : Constant  Value=2*pi*f
  w1 : Constant  Value=Vrif_M
  w4 : Constant  Value=Vdc_M
  tag scope: IbatM=global, PbatM=global, V_M=global, fase_M=global
  wires:
  Mux/1 -> [V_M]
  Proiezione a,b/3f I_f_rif/1(V_M1) -> Mux/1
  V_rif1/1 -> Media complessa/1(w), Integrator/1
  Proiezione a,b/3f I_f_rif/2(V_M2) -> Mux/2
  w1/1 -> Add/1
  Add/1 -> Proiezione a,b/3f I_f_rif/1(V_M_dq)
  Integrator/1 -> Media complessa/2(fase), [fase_M], Proiezione a,b/3f I_f_rif/2(Fase_inv)
  Proiezione a,b/3f I_f_rif/3(V_M3) -> Mux/3
  Media complessa/1(I_dc_d,q) -> PI Complesso/1(In1)
  [I_M_ab] -> Media complessa/3(I_a,b)
  [V_batM] -> Switch/2, Switch1/2
  Divide5/1 -> Switch/1
  Constant1/1 -> Switch1/3
  Constant/1 -> Switch1/1, Switch/3
  Switch/1 -> [IbatM]
  Switch1/1 -> Stop Simulation/1
  [P_M] -> Rate Limiter2/1
  w4/1 -> Divide5/2
  Rate Limiter2/1 -> [PbatM], Divide5/1
  PI Complesso/1(Out1) -> Add/2

== system RS_O_yalmip/DC PV ==
  Controlled Current Source : powerlib/Electrical Sources/Controlled Current Source  Initialize=on  Source_Type=DC  Amplitude=0  Phase=0  Frequency=0  Measurements=None
  Divide : Product  Inputs=*/
  Memory : Memory  X0=Vdc_2
  Rate Limiter3 : RateLimiter  RisingSlewLimit=1e6  FallingSlewLimit=-1e6  SampleTimeMode=inherited
  Ritardo_PLL2 : Subsystem
  Step1 : Step  Time=t3  Before=Ppv1  After=Ppv2  SampleTime=0
  Voltage Measurement : powerlib/Measurements/Voltage Measurement  PhasorSimulation=off  OutputType=Complex  PSBequivalent=0
  + : PMIOPort  Port=1  Side=Right
  - : PMIOPort  Port=2  Side=Right
  tag scope: P_pv=global
  wires:
  Voltage Measurement/1 -> Memory/1
  Step1/1 -> Ritardo_PLL2/1(P)
  Memory/1 -> Divide/2
  Divide/1 -> Controlled Current Source/1
  Ritardo_PLL2/1(g) -> Rate Limiter3/1
  Rate Limiter3/1 -> Divide/1, [P_pv]
  connections:
  Voltage Measurement/LConn1 -- +/RConn1 -- Controlled Current Source/RConn1
  Voltage Measurement/LConn2 -- -/RConn1 -- Controlled Current Source/LConn1

== system RS_O_yalmip/DC batterie1 ==
  Cbat : powerlib/Elements/Series RLC Branch  LConnTagsString=__new0  RConnTagsString=__new0  BranchType=C  Resistance=Rint  Inductance=0  SetiL0=off  InitialCurrent=0  Capacitance=Cint  Setx0=on  InitialVoltage=Vbat1  Measurements=None
  Controlled Current Source1 : powerlib/Electrical Sources/Controlled Current Source  Initialize=on  Source_Type=AC  Amplitude=0  Phase=0  Frequency=0  Measurements=None
  Controlled Current Source3 : powerlib/Electrical Sources/Controlled Current Source  Initialize=on  Source_Type=AC  Amplitude=0  Phase=0  Frequency=0  Measurements=None
  Divide : Product  Inputs=*/
  Divide1 : Product  Inputs=**
  Memory : Memory
  Memory1 : Memory
  Voltage Measurement : powerlib/Measurements/Voltage Measurement  PhasorSimulation=off  OutputType=Complex  PSBequivalent=0
  Voltage Measurement1 : powerlib/Measurements/Voltage Measurement  PhasorSimulation=off  OutputType=Complex  PSBequivalent=0
  bat + : PMIOPort  Tag=PMCPort  Port=1  Side=Left
  bat - : PMIOPort  Tag=PMCPort  Port=2  Side=Left
  V+ : PMIOPort  Tag=PMCPort  Port=3  Side=Right
  V- : PMIOPort  Tag=PMCPort  Port=4  Side=Right
  tag scope: V_bat1=global
  wires:
  Voltage Measurement1/1 -> Divide1/2, [V_bat1]
  [Ibat1] -> Memory1/1
  Memory1/1 -> Divide1/1, Controlled Current Source1/1
  Divide1/1 -> Divide/1
  Divide/1 -> Memory/1
  Memory/1 -> Controlled Current Source3/1
  Voltage Measurement/1 -> Divide/2
  connections:
  Cbat/LConn1 -- Controlled Current Source1/LConn1 -- Voltage Measurement1/LConn1 -- bat +/RConn1
  Cbat/RConn1 -- Controlled Current Source1/RConn1 -- Voltage Measurement1/LConn2 -- bat -/RConn1
  V+/RConn1 -- Voltage Measurement/LConn1 -- Controlled Current Source3/RConn1
  V-/RConn1 -- Controlled Current Source3/LConn1 -- Voltage Measurement/LConn2

== system RS_O_yalmip/DC batterie2 ==
  Cbat : powerlib/Elements/Series RLC Branch  LConnTagsString=__new0  RConnTagsString=__new0  BranchType=C  Resistance=Rint  Inductance=0  SetiL0=off  InitialCurrent=0  Capacitance=Cint  Setx0=on  InitialVoltage=Vbat2  Measurements=None
  Controlled Current Source1 : powerlib/Electrical Sources/Controlled Current Source  Initialize=on  Source_Type=AC  Amplitude=0  Phase=0  Frequency=0  Measurements=None
  Controlled Current Source3 : powerlib/Electrical Sources/Controlled Current Source  Initialize=on  Source_Type=AC  Amplitude=0  Phase=0  Frequency=0  Measurements=None
  Divide : Product  Inputs=*/
  Divide1 : Product  Inputs=**
  Memory : Memory
  Memory1 : Memory
  Voltage Measurement : powerlib/Measurements/Voltage Measurement  PhasorSimulation=off  OutputType=Complex  PSBequivalent=0
  Voltage Measurement1 : powerlib/Measurements/Voltage Measurement  PhasorSimulation=off  OutputType=Complex  PSBequivalent=0
  bat + : PMIOPort  Tag=PMCPort  Port=1  Side=Left
  bat - : PMIOPort  Tag=PMCPort  Port=2  Side=Left
  V+ : PMIOPort  Tag=PMCPort  Port=3  Side=Right
  V- : PMIOPort  Tag=PMCPort  Port=4  Side=Right
  tag scope: V_bat2=global
  wires:
  Voltage Measurement/1 -> Divide/2
  Memory/1 -> Controlled Current Source3/1
  Divide/1 -> Memory/1
  Divide1/1 -> Divide/1
  Memory1/1 -> Controlled Current Source1/1, Divide1/1
  [Ibat2] -> Memory1/1
  Voltage Measurement1/1 -> [V_bat2], Divide1/2
  connections:
  Controlled Current Source3/LConn1 -- V-/RConn1 -- Voltage Measurement/LConn2
  Voltage Measurement/LConn1 -- V+/RConn1 -- Controlled Current Source3/RConn1
  Controlled Current Source1/RConn1 -- Voltage Measurement1/LConn2 -- Cbat/RConn1 -- bat -/RConn1
  Voltage Measurement1/LConn1 -- Controlled Current Source1/LConn1 -- Cbat/LConn1 -- bat +/RConn1

== system RS_O_yalmip/DC batterieM ==
  Cbat : powerlib/Elements/Series RLC Branch  LConnTagsString=__new0  RConnTagsString=__new0  BranchType=C  Resistance=Rint  Inductance=0  SetiL0=off  InitialCurrent=0  Capacitance=Cint  Setx0=on  InitialVoltage=VbatM  Measurements=None
  Controlled Current Source1 : powerlib/Electrical Sources/Controlled Current Source  Initialize=on  Source_Type=AC  Amplitude=0  Phase=0  Frequency=0  Measurements=None
  Controlled Current Source3 : powerlib/Electrical Sources/Controlled Current Source  Initialize=on  Source_Type=AC  Amplitude=0  Phase=0  Frequency=0  Measurements=None
  Divide : Product  Inputs=*/
  Divide1 : Product  Inputs=**
  Memory : Memory
  Memory1 : Memory
  Voltage Measurement : powerlib/Measurements/Voltage Measurement  PhasorSimulation=off  OutputType=Complex  PSBequivalent=0
  Voltage Measurement1 : powerlib/Measurements/Voltage Measurement  PhasorSimulation=off  OutputType=Complex  PSBequivalent=0
  bat + : PMIOPort  Tag=PMCPort  Port=1  Side=Left
  bat - : PMIOPort  Tag=PMCPort  Port=2  Side=Left
  V+ : PMIOPort  Tag=PMCPort  Port=3  Side=Right
  V- : PMIOPort  Tag=PMCPort  Port=4  Side=Right
  tag scope: V_batM=global
  wires:
  Voltage Measurement/1 -> Divide/2
  Memory/1 -> Controlled Current Source3/1
  Divide/1 -> Memory/1
  Divide1/1 -> Divide/1
  Memory1/1 -> Controlled Current Source1/1, Divide1/1
  [IbatM] -> Memory1/1
  Voltage Measurement1/1 -> [V_batM], Divide1/2
  connections:
  Controlled Current Source3/LConn1 -- V-/RConn1 -- Voltage Measurement/LConn2
  Voltage Measurement/LConn1 -- V+/RConn1 -- Controlled Current Source3/RConn1
  Controlled Current Source1/RConn1 -- Voltage Measurement1/LConn2 -- Cbat/RConn1 -- bat -/RConn1
  Voltage Measurement1/LConn1 -- Controlled Current Source1/LConn1 -- Cbat/LConn1 -- bat +/RConn1

== system RS_O_yalmip/Inverter ID 1 ==
  C_f1 : powerlib/Elements/Series RLC Branch  LConnTagsString=__new0  RConnTagsString=__new0  BranchType=C  Resistance=Rc  Inductance=Lf  SetiL0=off  InitialCurrent=0  Capacitance=C1  Setx0=off  InitialVoltage=0  Measurements=None
  Controlled Current Source : powerlib/Electrical Sources/Controlled Current Source  Initialize=on  Source_Type=AC  Amplitude=0  Phase=0  Frequency=0  Measurements=None
  Controlled Current Source1 : powerlib/Electrical Sources/Controlled Current Source  Initialize=on  Source_Type=AC  Amplitude=0  Phase=0  Frequency=0  Measurements=None
  Controlled Current Source2 : powerlib/Electrical Sources/Controlled Current Source  Initialize=on  Source_Type=AC  Amplitude=0  Phase=0  Frequency=0  Measurements=None
  Current Measurement : powerlib/Measurements/Current Measurement  PhasorSimulation=off  OutputType=Complex  PSBequivalent=0
  DC Voltage Source : powerlib/Electrical Sources/DC Voltage Source  Amplitude=Vdc_1  Measurements=None
  Demux : Demux  Outputs=3
  Memory1 : Memory
  Series RLC Branch6 : powerlib/Elements/Series RLC Branch  LConnTagsString=__new0  RConnTagsString=__new0  BranchType=C  Resistance=Rc  Inductance=Lf  SetiL0=off  InitialCurrent=0  Capacitance=C1  Setx0=off  InitialVoltage=0  Measurements=None
  Series RLC Branch7 : powerlib/Elements/Series RLC Branch  LConnTagsString=__new0  RConnTagsString=__new0  BranchType=C  Resistance=Rc  Inductance=Lf  SetiL0=off  InitialCurrent=0  Capacitance=C1  Setx0=off  InitialVoltage=0  Measurements=None
  Subsystem2 : Subsystem
  Three-Phase V-I Measurement : powerlib/Measurements/Three-Phase V-I Measurement  VoltageMeasurement=phase-to-phase  SetLabelV=off  LabelV=Vabc  Vpu=off  VpuLL=off  CurrentMeasurement=no  SetLabelI=off  LabelI=Iabc  Ipu=off  Pbase=100e6  Vbase=500e3  OutputType=Complex  PhasorSimulation=off  PSBequivalent=0
  1 : PMIOPort  Tag=PMCPort  Port=1  Side=Right
  2 : PMIOPort  Tag=PMCPort  Port=2  Side=Right
  3 : PMIOPort  Tag=PMCPort  Port=3  Side=Right
  V+ : PMIOPort  Tag=PMCPort  Port=4  Side=Left
  V- : PMIOPort  Tag=PMCPort  Port=5  Side=Left
  tag scope: Idc1=global, V_1_abc=global
  wires:
  Subsystem2/1(V_f) -> [V_1_abc]
  Three-Phase V-I Measurement/1 -> Subsystem2/1(V_c)
  Demux/2 -> Controlled Current Source1/1
  Demux/3 -> Controlled Current Source2/1
  Demux/1 -> Controlled Current Source/1
  [I_1] -> Memory1/1
  Memory1/1 -> Demux/1
  Current Measurement/1 -> [Idc1]
  connections:
  V-/RConn1 -- DC Voltage Source/LConn1
  V+/RConn1 -- Current Measurement/RConn1
  C_f1/RConn1 -- Series RLC Branch6/RConn1 -- Controlled Current Source2/LConn1 -- Controlled Current Source1/LConn1 -- Controlled Current Source/LConn1 -- Series RLC Branch7/RConn1
  Controlled Current Source/RConn1 -- Three-Phase V-I Measurement/LConn1
  Controlled Current Source2/RConn1 -- Three-Phase V-I Measurement/LConn3
  Three-Phase V-I Measurement/LConn2 -- Controlled Current Source1/RConn1
  Three-Phase V-I Measurement/RConn2 -- Series RLC Branch7/LConn1 -- 2/RConn1
  1/RConn1 -- Series RLC Branch6/LConn1 -- Three-Phase V-I Measurement/RConn1
  3/RConn1 -- Three-Phase V-I Measurement/RConn3 -- C_f1/LConn1
  Current Measurement/LConn1 -- DC Voltage Source/RConn1

== system RS_O_yalmip/Inverter ID 2 ==
  C_f2 : powerlib/Elements/Series RLC Branch  LConnTagsString=__new0  RConnTagsString=__new0  BranchType=C  Resistance=Rc  Inductance=Lf  SetiL0=off  InitialCurrent=0  Capacitance=C2  Setx0=off  InitialVoltage=0  Measurements=None
  Controlled Current Source : powerlib/Electrical Sources/Controlled Current Source  Initialize=on  Source_Type=AC  Amplitude=0  Phase=0  Frequency=0  Measurements=None
  Controlled Current Source1 : powerlib/Electrical Sources/Controlled Current Source  Initialize=on  Source_Type=AC  Amplitude=0  Phase=0  Frequency=0  Measurements=None
  Controlled Current Source2 : powerlib/Electrical Sources/Controlled Current Source  Initialize=on  Source_Type=AC  Amplitude=0  Phase=0  Frequency=0  Measurements=None
  Current Measurement : powerlib/Measurements/Current Measurement  PhasorSimulation=off  OutputType=Complex  PSBequivalent=0
  DC Voltage Source : powerlib/Electrical Sources/DC Voltage Source  Amplitude=Vdc_2  Measurements=None
  Demux : Demux  Outputs=3
  Memory1 : Memory
  Series RLC Branch6 : powerlib/Elements/Series RLC Branch  LConnTagsString=__new0  RConnTagsString=__new0  BranchType=C  Resistance=Rc  Inductance=Lf  SetiL0=off  InitialCurrent=0  Capacitance=C2  Setx0=off  InitialVoltage=0  Measurements=None
  Series RLC Branch7 : powerlib/Elements/Series RLC Branch  LConnTagsString=__new0  RConnTagsString=__new0  BranchType=C  Resistance=Rc  Inductance=Lf  SetiL0=off  InitialCurrent=0  Capacitance=C2  Setx0=off  InitialVoltage=0  Measurements=None
  Subsystem2 : Subsystem
  Three-Phase V-I Measurement : powerlib/Measurements/Three-Phase V-I Measurement  VoltageMeasurement=phase-to-phase  SetLabelV=off  LabelV=Vabc  Vpu=off  VpuLL=off  CurrentMeasurement=no  SetLabelI=off  LabelI=Iabc  Ipu=off  Pbase=100e6  Vbase=500e3  OutputType=Complex  PhasorSimulation=off  PSBequivalent=0
  1 : PMIOPort  Tag=PMCPort  Port=1  Side=Right
  2 : PMIOPort  Tag=PMCPort  Port=2  Side=Right
  3 : PMIOPort  Tag=PMCPort  Port=3  Side=Right
  V+ : PMIOPort  Tag=PMCPort  Port=4  Side=Left
  V- : PMIOPort  Tag=PMCPort  Port=5  Side=Left
  tag scope: Idc2=global, V_2_abc=global
  wires:
  Memory1/1 -> Demux/1
  [I_2] -> Memory1/1
  Demux/1 -> Controlled Current Source/1
  Demux/3 -> Controlled Current Source2/1
  Demux/2 -> Controlled Current Source1/1
  Three-Phase V-I Measurement/1 -> Subsystem2/1(V_c)
  Subsystem2/1(V_f) -> [V_2_abc]
  Current Measurement/1 -> [Idc2]
  connections:
  C_f2/LConn1 -- Three-Phase V-I Measurement/RConn3 -- 3/RConn1
  Three-Phase V-I Measurement/RConn1 -- Series RLC Branch6/LConn1 -- 1/RConn1
  2/RConn1 -- Series RLC Branch7/LConn1 -- Three-Phase V-I Measurement/RConn2
  Three-Phase V-I Measurement/LConn2 -- Controlled Current Source1/RConn1
  Controlled Current Source2/RConn1 -- Three-Phase V-I Measurement/LConn3
  Controlled Current Source/RConn1 -- Three-Phase V-I Measurement/LConn1
  Series RLC Branch7/RConn1 -- Series RLC Branch6/RConn1 -- Controlled Current Source/LConn1 -- Controlled Current Source1/LConn1 -- Controlled Current Source2/LConn1 -- C_f2/RConn1
  Current Measurement/LConn1 -- DC Voltage Source/RConn1
  V+/RConn1 -- Current Measurement/RConn1
  V-/RConn1 -- DC Voltage Source/LConn1

== system RS_O_yalmip/Inverter ID M ==
  Controlled Voltage Source : powerlib/Electrical Sources/Controlled Voltage Source  Initialize=on  Source_Type=AC  Amplitude=0  Phase=0  Frequency=0  Measurements=None
  Controlled Voltage Source1 : powerlib/Electrical Sources/Controlled Voltage Source  Initialize=on  Source_Type=AC  Amplitude=0  Phase=0  Frequency=0  Measurements=None
  Controlled Voltage Source2 : powerlib/Electrical Sources/Controlled Voltage Source  Initialize=on  Source_Type=AC  Amplitude=0  Phase=0  Frequency=0  Measurements=None
  Current Measurement : powerlib/Measurements/Current Measurement  PhasorSimulation=off  OutputType=Complex  PSBequivalent=0
  DC Voltage Source : powerlib/Electrical Sources/DC Voltage Source  Amplitude=Vdc_M  Measurements=None
  Demux : Demux  Outputs=3
  Memory1 : Memory
  Three-Phase V-I Measurement : powerlib/Measurements/Three-Phase V-I Measurement  VoltageMeasurement=no  SetLabelV=off  LabelV=Vabc  Vpu=off  VpuLL=off  CurrentMeasurement=yes  SetLabelI=off  LabelI=Iabc  Ipu=off  Pbase=100e6  Vbase=500e3  OutputType=Complex  PhasorSimulation=off  PSBequivalent=0
  1 : PMIOPort  Tag=PMCPort  Port=1  Side=Right
  2 : PMIOPort  Tag=PMCPort  Port=2  Side=Right
  3 : PMIOPort  Tag=PMCPort  Port=3  Side=Right
  V+ : PMIOPort  Tag=PMCPort  Port=4  Side=Left
  V- : PMIOPort  Tag=PMCPort  Port=5  Side=Left
  tag scope: I_M_abc=global, IdcM=global
  wires:
  Three-Phase V-I Measurement/1 -> [I_M_abc]
  Demux/3 -> Controlled Voltage Source2/1
  Demux/2 -> Controlled Voltage Source1/1
  Demux/1 -> Controlled Voltage Source/1
  [V_M] -> Memory1/1
  Memory1/1 -> Demux/1
  Current Measurement/1 -> [IdcM]
  connections:
  Three-Phase V-I Measurement/LConn1 -- Controlled Voltage Source/RConn1
  Three-Phase V-I Measurement/LConn3 -- Controlled Voltage Source2/RConn1
  Three-Phase V-I Measurement/LConn2 -- Controlled Voltage Source1/RConn1
  Three-Phase V-I Measurement/RConn1 -- 1/RConn1
  Three-Phase V-I Measurement/RConn2 -- 2/RConn1
  Three-Phase V-I Measurement/RConn3 -- 3/RConn1
  Controlled Voltage Source1/LConn1 -- Controlled Voltage Source/LConn1 -- Controlled Voltage Source2/LConn1
  V-/RConn1 -- DC Voltage Source/LConn1
  Current Measurement/LConn1 -- DC Voltage Source/RConn1
  V+/RConn1 -- Current Measurement/RConn1
